simulink model "control"  (R2021b)
settings: Solver=FixedStepDiscrete  StartTime=0.0  StopTime=inf  FixedStep=0.02  RelTol=1e-3
undefined symbols (not defined in the file): Radix
libraries: dspstat3 x6, simulink x2, dspxfrm3 x1, dspsigops x1, simulink_extras x1
settings Model: Creator=jekyll  LastModifiedBy=jekyll
settings OptimizationCC: DefaultParameterBehavior=Inlined  EnhancedBackFolding=on  PassReuseOutputArgsAs=Individual arguments  ZeroExternalMemoryAtStartup=off  ZeroInternalMemoryAtStartup=off  OptimizeBlockOrder=speed  DifferentSizesBufferReuse=on  OptimizationCustomize=off  EfficientTunableParamExpr=on
settings DebuggingCC: ParameterTunabilityLossMsg=error  UnconnectedInputMsg=none  UnconnectedOutputMsg=none  UnconnectedLineMsg=none
settings ModelReferenceCC: EnableRefExpFcnMdlSchedulingChecks=off
settings SFSimCC: MATLABDynamicMemAlloc=off
settings RTWCC: Description=Embedded Coder  SystemTargetFile=ert.tlc  GenCodeOnly=on  TemplateMakefile=ert_default_tmf  CustomHeaderCode=#include <emscripten/emscripten.h>  GPUComputeCapability=5.0  DLArmComputeVersion=20.02.1
settings CodeAppCC: ForceParamTrailComments=on  IgnoreCustomStorageClasses=off  OperatorAnnotations=on  SimulinkDataObjDesc=on  SFDataObjDesc=on  InsertBlockDesc=on
settings ERTTargetCC: TargetLangStandard=C99 (ISO)  GenerateSampleERTMain=on  InlinedParameterPlacement=NonHierarchical  ERTCustomFileTemplate=example_file_process.tlc

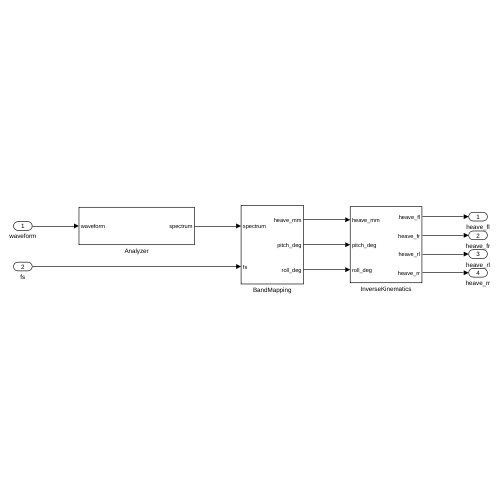
[thumbnail: Simulink's stored preview of the top-level diagram]
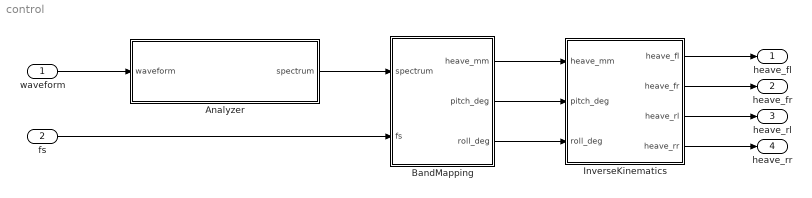
== system control ==
  waveform : Inport  PortDimensions=512
  fs : Inport  Port=2
  Analyzer : Subsystem
  BandMapping : Subsystem
  InverseKinematics : Subsystem
  heave_fl : Outport
  heave_fr : Outport  Port=2
  heave_rl : Outport  Port=3
  heave_rr : Outport  Port=4
  wires:
  waveform/1 -> Analyzer/1(waveform)
  Analyzer/1(spectrum) -> BandMapping/1(spectrum)
  fs/1 -> BandMapping/2(fs)
  BandMapping/3(roll_deg) -> InverseKinematics/3(roll_deg)
  InverseKinematics/1(heave_fl) -> heave_fl/1
  InverseKinematics/2(heave_fr) -> heave_fr/1
  InverseKinematics/3(heave_rl) -> heave_rl/1
  InverseKinematics/4(heave_rr) -> heave_rr/1
  BandMapping/1(heave_mm) -> InverseKinematics/1(heave_mm)
  BandMapping/2(pitch_deg) -> InverseKinematics/2(pitch_deg)

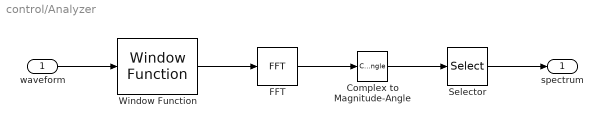
== system control/Analyzer ==
  waveform : Inport
  Complex to Magnitude-Angle : ComplexToMagnitudeAngle  Output=Magnitude
  FFT : dspxfrm3/FFT  FFTImplementation=Radix-2  CompMethod=Table lookup  TableOpt=NEW  TableOptActive=Speed  BitRevOrder=off  Normalize=on  InheritFFTLength=off  FFTLength=512  WrapInput=on  roundingMode=Floor  overflowMode=off  firstCoeffDataTypeStr=Inherit: Same word length as input  firstCoeffLastDataTypeStr=Inherit: Same word length as input  outputMin=[]  outputMax=[]
  Selector : Selector  IndexMode=Zero-based  InputPortWidth=512  IndexOptions=Index vector (dialog)  Indices=[0:255]  OutputSizes=1
  Window Function : dspsigops/Window Function  winmode=Apply window to input  wintype=Hann  sampmode=Continuous  samptime=1  N=64  Rs=50  beta=10  winsamp=Symmetric  UserWindow=hamming  OptParams=off  UserParams={'symmetric'}  dataType=double  isSigned=on  wordLen=16  udDataType=sfix(16)  fracBitsMode=Best precision  numFracBits=15  roundingMode=Floor  overflowMode=off  numSidelobes=4  sidelobeLevel=-30
      settings: SourceProductBaseCode=DS
  spectrum : Outport
  wires:
  Window Function/1 -> FFT/1
  FFT/1 -> Complex to Magnitude-Angle/1
  Complex to Magnitude-Angle/1 -> Selector/1
  waveform/1 -> Window Function/1
  Selector/1 -> spectrum/1

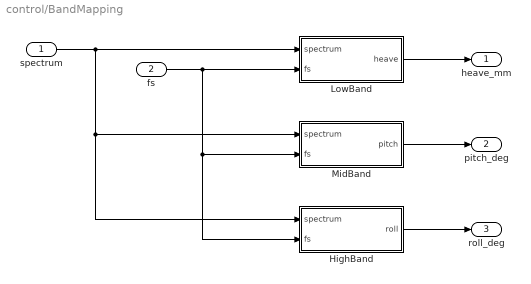
== system control/BandMapping ==
  spectrum : Inport
  fs : Inport  Port=2
  HighBand : Subsystem
  LowBand : Subsystem
  MidBand : Subsystem
  heave_mm : Outport
  pitch_deg : Outport  Port=2
  roll_deg : Outport  Port=3
  wires:
  spectrum/1 -> LowBand/1(spectrum), HighBand/1(spectrum), MidBand/1(spectrum)
  fs/1 -> HighBand/2(fs), MidBand/2(fs), LowBand/2(fs)
  LowBand/1(heave) -> heave_mm/1
  MidBand/1(pitch) -> pitch_deg/1
  HighBand/1(roll) -> roll_deg/1

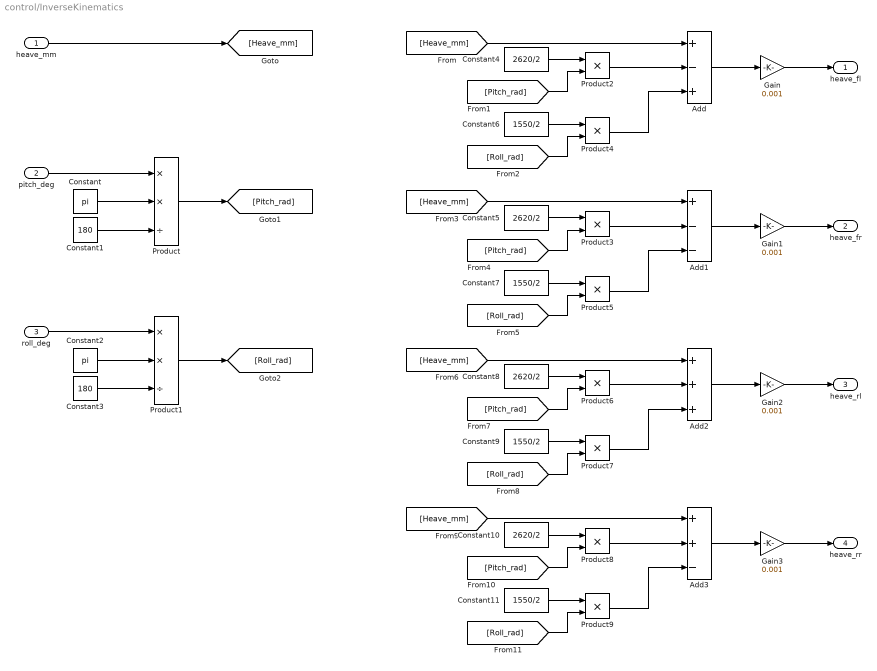
== system control/InverseKinematics ==
  heave_mm : Inport
  pitch_deg : Inport  Port=2
  roll_deg : Inport  Port=3
  Add : Sum  Inputs=+-+
  Add1 : Sum  Inputs=+--
  Add2 : Sum  Inputs=+++
  Add3 : Sum  Inputs=++-
  Constant : Constant  Value=pi
  Constant1 : Constant  Value=180
  Constant{4..5,8,10} (4 alike) : Constant  Value=2620/2
  Constant{6..7,9,11} (4 alike) : Constant  Value=1550/2
  Constant2 : Constant  Value=pi
  Constant3 : Constant  Value=180
  Gain{,1..3} (4 alike) : Gain  Gain=0.001
  Product : Product  Inputs=**/
  Product1 : Product  Inputs=**/
  Product{2..9} (8 alike) : Product
  heave_fl : Outport
  heave_fr : Outport  Port=2
  heave_rl : Outport  Port=3
  heave_rr : Outport  Port=4
  wires:
  Add/1 -> Gain/1
  pitch_deg/1 -> Product/1
  Constant/1 -> Product/2
  Constant1/1 -> Product/3
  Constant3/1 -> Product1/3
  Constant2/1 -> Product1/2
  roll_deg/1 -> Product1/1
  heave_mm/1 -> [Heave_mm]
  Product/1 -> [Pitch_rad]
  Product1/1 -> [Roll_rad]
  [Heave_mm] -> Add/1
  Product2/1 -> Add/2
  Constant4/1 -> Product2/1
  [Pitch_rad] -> Product2/2
  [Roll_rad] -> Product4/2
  Product4/1 -> Add/3
  Constant6/1 -> Product4/1
  Constant7/1 -> Product5/1
  Product5/1 -> Add1/3
  [Roll_rad] -> Product5/2
  [Pitch_rad] -> Product3/2
  Constant5/1 -> Product3/1
  Product3/1 -> Add1/2
  [Heave_mm] -> Add1/1
  Add1/1 -> Gain1/1
  Add2/1 -> Gain2/1
  [Heave_mm] -> Add2/1
  Product6/1 -> Add2/2
  Constant8/1 -> Product6/1
  [Pitch_rad] -> Product6/2
  [Roll_rad] -> Product7/2
  Product7/1 -> Add2/3
  Constant9/1 -> Product7/1
  Constant11/1 -> Product9/1
  Product9/1 -> Add3/3
  [Roll_rad] -> Product9/2
  [Pitch_rad] -> Product8/2
  Constant10/1 -> Product8/1
  Product8/1 -> Add3/2
  [Heave_mm] -> Add3/1
  Add3/1 -> Gain3/1
  Gain/1 -> heave_fl/1
  Gain1/1 -> heave_fr/1
  Gain2/1 -> heave_rl/1
  Gain3/1 -> heave_rr/1

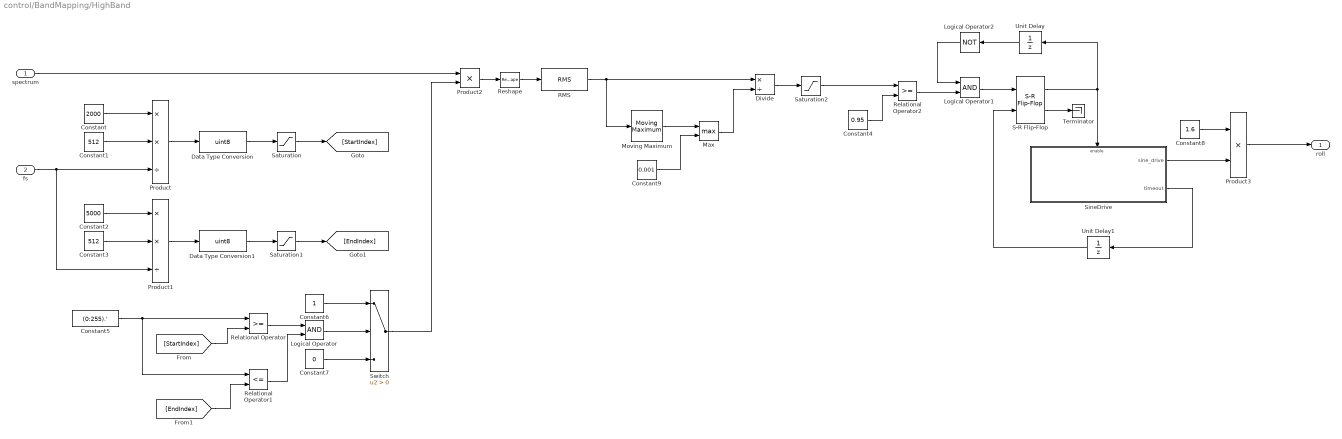
== system control/BandMapping/HighBand ==
  spectrum : Inport
  fs : Inport  Port=2
  Constant : Constant  Value=2000
  Constant1 : Constant  Value=512
  Constant2 : Constant  Value=5000
  Constant3 : Constant  Value=512
  Constant4 : Constant  Value=0.95
  Constant5 : Constant  Value=(0:255).'
  Constant6 : Constant
  Constant7 : Constant  Value=0
  Constant8 : Constant  Value=1.6
  Constant9 : Constant  Value=0.001
  Data Type Conversion : DataTypeConversion  OutDataTypeStr=uint8  RndMeth=Nearest
  Data Type Conversion1 : DataTypeConversion  OutDataTypeStr=uint8  RndMeth=Nearest
  Divide : Product  Inputs=*/
  Logical Operator : Logic  AllPortsSameDT=off  OutDataTypeStr=boolean
  Logical Operator1 : Logic  AllPortsSameDT=off  OutDataTypeStr=boolean
  Logical Operator2 : Logic  Operator=NOT  AllPortsSameDT=off  OutDataTypeStr=boolean
  Max : MinMax  Function=max  Inputs=2
  Moving Maximum : dspstat3/Moving Maximum  SpecifyWindowLength=on  WindowLength=100  SimulateUsing=Code generation
      settings: SourceProductBaseCode=DS
  Product : Product  Inputs=**/
  Product1 : Product  Inputs=**/
  Product2 : Product
  Product3 : Product
  RMS : dspstat3/RMS  run=off  directionMode=Entire input  dimension=1  InputProcessing=Columns as channels (frame based)  reset_popup=None
  Relational Operator : RelationalOperator  OutDataTypeStr=boolean  RndMeth=Simplest
  Relational Operator1 : RelationalOperator  Operator=<=  OutDataTypeStr=boolean  RndMeth=Simplest
  Relational Operator2 : RelationalOperator  OutDataTypeStr=boolean  RndMeth=Simplest
  Reshape : Reshape
  S-R Flip-Flop : simulink_extras/Flip Flops/S-R Flip-Flop  initial_condition=0
  Saturation : Saturate  UpperLimit=255  LowerLimit=0
  Saturation1 : Saturate  UpperLimit=255  LowerLimit=0
  Saturation2 : Saturate  UpperLimit=1  LowerLimit=0
  SineDrive : Subsystem  TreatAsAtomicUnit=on
  Switch : Switch  Criteria=u2 > Threshold
  Terminator : Terminator
  Unit Delay : UnitDelay  SampleTime=-1  HasFrameUpgradeWarning=on
  Unit Delay1 : UnitDelay  SampleTime=-1  HasFrameUpgradeWarning=on
  roll : Outport
  wires:
  spectrum/1 -> Product2/1
  Constant/1 -> Product/1
  Constant1/1 -> Product/2
  fs/1 -> Product/3, Product1/3
  Constant3/1 -> Product1/2
  Constant2/1 -> Product1/1
  Product/1 -> Data Type Conversion/1
  Product1/1 -> Data Type Conversion1/1
  Data Type Conversion/1 -> Saturation/1
  Data Type Conversion1/1 -> Saturation1/1
  Constant5/1 -> Relational Operator1/1, Relational Operator/1
  Saturation/1 -> [StartIndex]
  Saturation1/1 -> [EndIndex]
  [StartIndex] -> Relational Operator/2
  [EndIndex] -> Relational Operator1/2
  Relational Operator/1 -> Logical Operator/1
  Relational Operator1/1 -> Logical Operator/2
  Logical Operator/1 -> Switch/2
  Constant6/1 -> Switch/1
  Constant7/1 -> Switch/3
  Switch/1 -> Product2/2
  Product2/1 -> Reshape/1
  Reshape/1 -> RMS/1
  Product3/1 -> roll/1
  Constant4/1 -> Relational Operator2/2
  Logical Operator1/1 -> S-R Flip-Flop/1
  Relational Operator2/1 -> Logical Operator1/2
  Unit Delay/1 -> Logical Operator2/1
  S-R Flip-Flop/1 -> Unit Delay/1, SineDrive/Enable
  S-R Flip-Flop/2 -> Terminator/1
  Logical Operator2/1 -> Logical Operator1/1
  SineDrive/2(timeout) -> Unit Delay1/1
  Unit Delay1/1 -> S-R Flip-Flop/2
  RMS/1 -> Moving Maximum/1, Divide/1
  Moving Maximum/1 -> Max/1
  Max/1 -> Divide/2
  Constant9/1 -> Max/2
  Divide/1 -> Saturation2/1
  Saturation2/1 -> Relational Operator2/1
  SineDrive/1(sine_drive) -> Product3/2
  Constant8/1 -> Product3/1

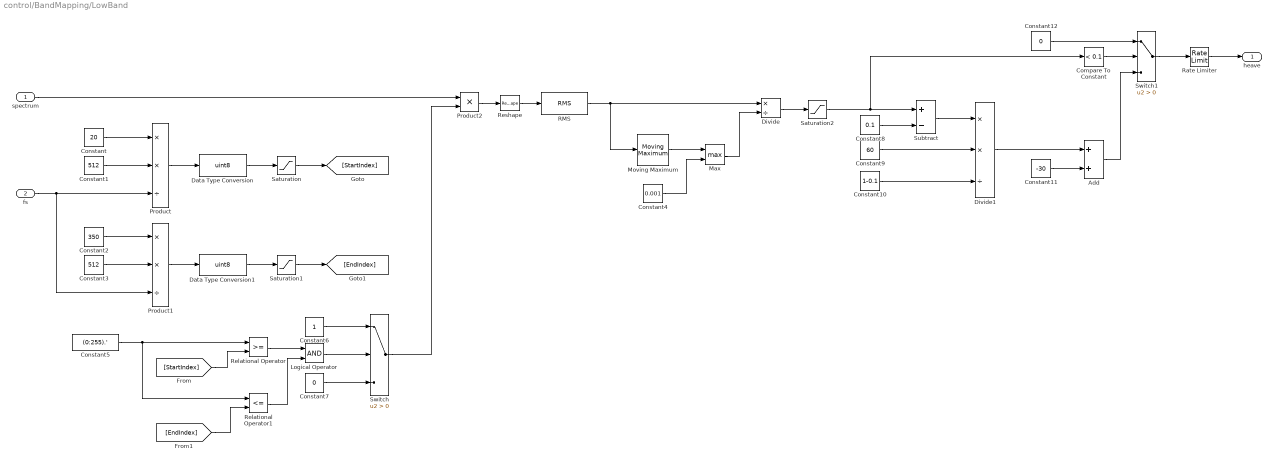
== system control/BandMapping/LowBand ==
  spectrum : Inport
  fs : Inport  Port=2
  Add : Sum
  Compare To Constant : simulink/Logic and Bit Operations/Compare To Constant  relop=<  const=0.1  OutDataTypeStr=boolean
  Constant : Constant  Value=20
  Constant1 : Constant  Value=512
  Constant10 : Constant  Value=1-0.1
  Constant11 : Constant  Value=-30
  Constant12 : Constant  Value=0
  Constant2 : Constant  Value=350
  Constant3 : Constant  Value=512
  Constant4 : Constant  Value=0.001
  Constant5 : Constant  Value=(0:255).'
  Constant6 : Constant
  Constant7 : Constant  Value=0
  Constant8 : Constant  Value=0.1
  Constant9 : Constant  Value=60
  Data Type Conversion : DataTypeConversion  OutDataTypeStr=uint8  RndMeth=Nearest
  Data Type Conversion1 : DataTypeConversion  OutDataTypeStr=uint8  RndMeth=Nearest
  Divide : Product  Inputs=*/
  Divide1 : Product  Inputs=**/
  Logical Operator : Logic  AllPortsSameDT=off  OutDataTypeStr=boolean
  Max : MinMax  Function=max  Inputs=2
  Moving Maximum : dspstat3/Moving Maximum  SpecifyWindowLength=on  WindowLength=100  SimulateUsing=Code generation
      settings: SourceProductBaseCode=DS
  Product : Product  Inputs=**/
  Product1 : Product  Inputs=**/
  Product2 : Product
  RMS : dspstat3/RMS  run=off  directionMode=Entire input  dimension=1  InputProcessing=Columns as channels (frame based)  reset_popup=None
  Rate Limiter : RateLimiter  RisingSlewLimit=30/1  FallingSlewLimit=-30/1  SampleTimeMode=inherited
  Relational Operator : RelationalOperator  OutDataTypeStr=boolean  RndMeth=Simplest
  Relational Operator1 : RelationalOperator  Operator=<=  OutDataTypeStr=boolean  RndMeth=Simplest
  Reshape : Reshape
  Saturation : Saturate  UpperLimit=255  LowerLimit=0
  Saturation1 : Saturate  UpperLimit=255  LowerLimit=0
  Saturation2 : Saturate  UpperLimit=1  LowerLimit=0
  Subtract : Sum  Inputs=+-
  Switch : Switch  Criteria=u2 > Threshold
  Switch1 : Switch  Criteria=u2 > Threshold
  heave : Outport
  wires:
  spectrum/1 -> Product2/1
  Constant/1 -> Product/1
  Constant1/1 -> Product/2
  fs/1 -> Product/3, Product1/3
  Constant3/1 -> Product1/2
  Constant2/1 -> Product1/1
  Product/1 -> Data Type Conversion/1
  Product1/1 -> Data Type Conversion1/1
  Data Type Conversion/1 -> Saturation/1
  Data Type Conversion1/1 -> Saturation1/1
  RMS/1 -> Divide/1, Moving Maximum/1
  Moving Maximum/1 -> Max/1
  Constant4/1 -> Max/2
  Max/1 -> Divide/2
  Divide/1 -> Saturation2/1
  Constant5/1 -> Relational Operator1/1, Relational Operator/1
  Saturation/1 -> [StartIndex]
  Saturation1/1 -> [EndIndex]
  [StartIndex] -> Relational Operator/2
  [EndIndex] -> Relational Operator1/2
  Relational Operator/1 -> Logical Operator/1
  Relational Operator1/1 -> Logical Operator/2
  Logical Operator/1 -> Switch/2
  Constant6/1 -> Switch/1
  Constant7/1 -> Switch/3
  Switch/1 -> Product2/2
  Product2/1 -> Reshape/1
  Reshape/1 -> RMS/1
  Constant8/1 -> Subtract/2
  Subtract/1 -> Divide1/1
  Constant9/1 -> Divide1/2
  Constant10/1 -> Divide1/3
  Divide1/1 -> Add/1
  Constant11/1 -> Add/2
  Rate Limiter/1 -> heave/1
  Saturation2/1 -> Compare To Constant/1, Subtract/1
  Compare To Constant/1 -> Switch1/2
  Constant12/1 -> Switch1/1
  Switch1/1 -> Rate Limiter/1
  Add/1 -> Switch1/3

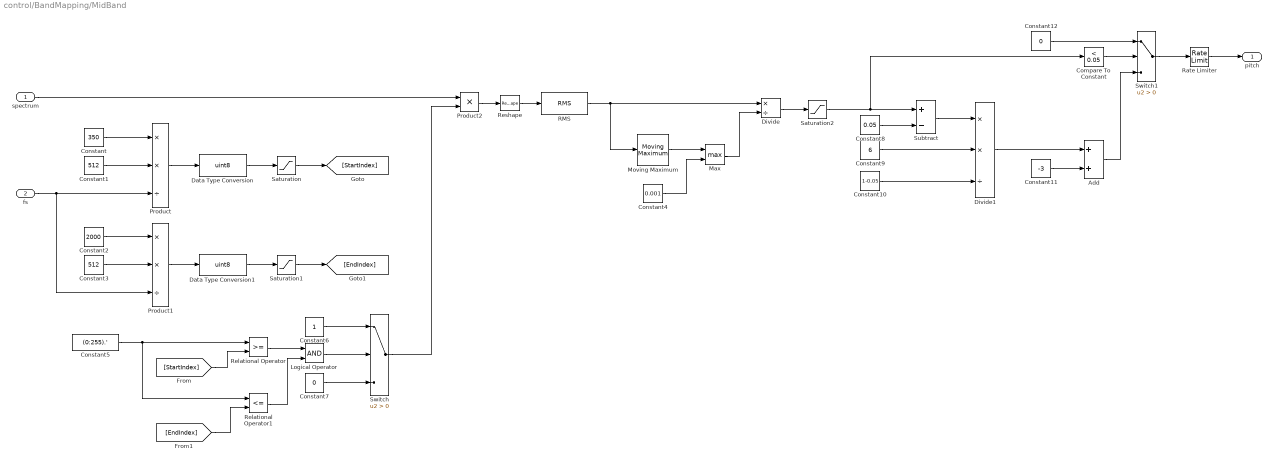
== system control/BandMapping/MidBand ==
  spectrum : Inport
  fs : Inport  Port=2
  Add : Sum
  Compare To Constant : simulink/Logic and Bit Operations/Compare To Constant  relop=<  const=0.05  OutDataTypeStr=boolean
  Constant : Constant  Value=350
  Constant1 : Constant  Value=512
  Constant10 : Constant  Value=1-0.05
  Constant11 : Constant  Value=-3
  Constant12 : Constant  Value=0
  Constant2 : Constant  Value=2000
  Constant3 : Constant  Value=512
  Constant4 : Constant  Value=0.001
  Constant5 : Constant  Value=(0:255).'
  Constant6 : Constant
  Constant7 : Constant  Value=0
  Constant8 : Constant  Value=0.05
  Constant9 : Constant  Value=6
  Data Type Conversion : DataTypeConversion  OutDataTypeStr=uint8  RndMeth=Nearest
  Data Type Conversion1 : DataTypeConversion  OutDataTypeStr=uint8  RndMeth=Nearest
  Divide : Product  Inputs=*/
  Divide1 : Product  Inputs=**/
  Logical Operator : Logic  AllPortsSameDT=off  OutDataTypeStr=boolean
  Max : MinMax  Function=max  Inputs=2
  Moving Maximum : dspstat3/Moving Maximum  SpecifyWindowLength=on  WindowLength=100  SimulateUsing=Code generation
      settings: SourceProductBaseCode=DS
  Product : Product  Inputs=**/
  Product1 : Product  Inputs=**/
  Product2 : Product
  RMS : dspstat3/RMS  run=off  directionMode=Entire input  dimension=1  InputProcessing=Columns as channels (frame based)  reset_popup=None
  Rate Limiter : RateLimiter  RisingSlewLimit=3/1  FallingSlewLimit=-3/1  SampleTimeMode=inherited
  Relational Operator : RelationalOperator  OutDataTypeStr=boolean  RndMeth=Simplest
  Relational Operator1 : RelationalOperator  Operator=<=  OutDataTypeStr=boolean  RndMeth=Simplest
  Reshape : Reshape
  Saturation : Saturate  UpperLimit=255  LowerLimit=0
  Saturation1 : Saturate  UpperLimit=255  LowerLimit=0
  Saturation2 : Saturate  UpperLimit=1  LowerLimit=0
  Subtract : Sum  Inputs=+-
  Switch : Switch  Criteria=u2 > Threshold
  Switch1 : Switch  Criteria=u2 > Threshold
  pitch : Outport
  wires:
  Add/1 -> Switch1/3
  Switch1/1 -> Rate Limiter/1
  Constant12/1 -> Switch1/1
  Compare To Constant/1 -> Switch1/2
  Saturation2/1 -> Subtract/1, Compare To Constant/1
  Rate Limiter/1 -> pitch/1
  Constant11/1 -> Add/2
  Divide1/1 -> Add/1
  Constant10/1 -> Divide1/3
  Constant9/1 -> Divide1/2
  Subtract/1 -> Divide1/1
  Constant8/1 -> Subtract/2
  Reshape/1 -> RMS/1
  Product2/1 -> Reshape/1
  Switch/1 -> Product2/2
  Constant7/1 -> Switch/3
  Constant6/1 -> Switch/1
  Logical Operator/1 -> Switch/2
  Relational Operator1/1 -> Logical Operator/2
  Relational Operator/1 -> Logical Operator/1
  [EndIndex] -> Relational Operator1/2
  [StartIndex] -> Relational Operator/2
  Saturation1/1 -> [EndIndex]
  Saturation/1 -> [StartIndex]
  Constant5/1 -> Relational Operator/1, Relational Operator1/1
  Divide/1 -> Saturation2/1
  Max/1 -> Divide/2
  Constant4/1 -> Max/2
  Moving Maximum/1 -> Max/1
  RMS/1 -> Moving Maximum/1, Divide/1
  Data Type Conversion1/1 -> Saturation1/1
  Data Type Conversion/1 -> Saturation/1
  Product1/1 -> Data Type Conversion1/1
  Product/1 -> Data Type Conversion/1
  Constant2/1 -> Product1/1
  Constant3/1 -> Product1/2
  fs/1 -> Product1/3, Product/3
  Constant1/1 -> Product/2
  Constant/1 -> Product/1
  spectrum/1 -> Product2/1

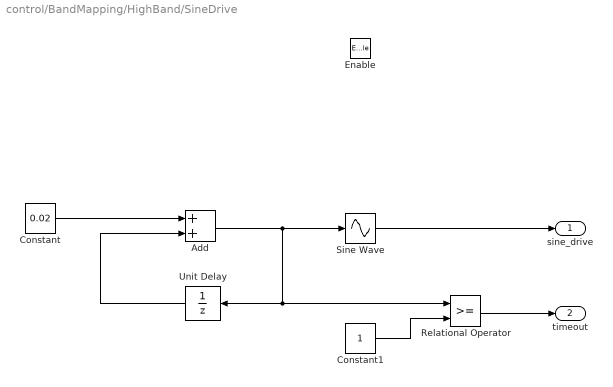
== system control/BandMapping/HighBand/SineDrive ==
  Enable : EnablePort  StatesWhenEnabling=reset
  Add : Sum
  Constant : Constant  Value=0.02
  Constant1 : Constant
  Relational Operator : RelationalOperator  OutDataTypeStr=boolean  RndMeth=Simplest
  Sine Wave : Sin  TimeSource=Use external signal  Frequency=2*pi  SampleTime=0
  Unit Delay : UnitDelay  SampleTime=-1  HasFrameUpgradeWarning=on
  sine_drive : Outport  OutputWhenDisabled=reset  InitialOutput=0
  timeout : Outport  Port=2  OutputWhenDisabled=reset  InitialOutput=0
  wires:
  Sine Wave/1 -> sine_drive/1
  Constant/1 -> Add/1
  Add/1 -> Relational Operator/1, Unit Delay/1, Sine Wave/1
  Unit Delay/1 -> Add/2
  Constant1/1 -> Relational Operator/2
  Relational Operator/1 -> timeout/1
